simulink model "lab_2_n_4_Liza"  (R2021b)
settings: Solver=VariableStepAuto  StartTime=0.0  StopTime=100.0  RelTol=1e-3
libraries: simulink x1
settings Model: Creator=peter  LastModifiedBy=peter

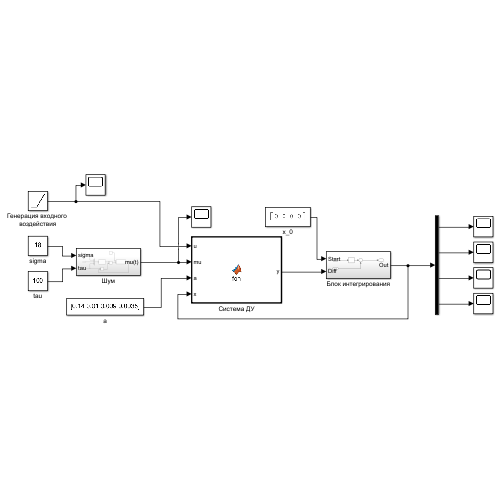
[thumbnail: Simulink's stored preview of the top-level diagram]
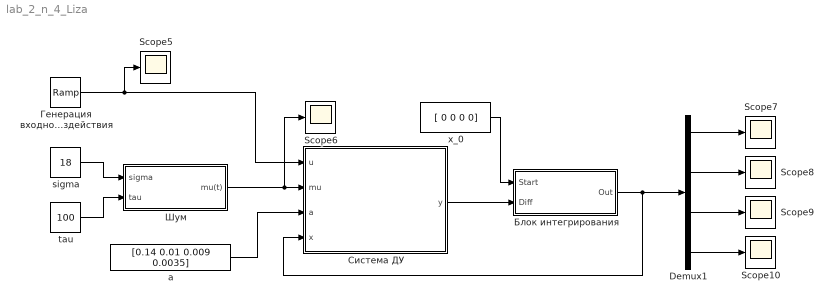
== system lab_2_n_4_Liza ==
  Demux1 : Demux
  Scope{5..10} (6 alike) : Scope
  a : Constant  Value=[0.14 0.01 0.009 0.0035]
  sigma : Constant  Value=18
  tau : Constant  Value=100
  x_0 : Constant  Value=[ 0 0 0 0]
  Блок интегрирования : Subsystem
  Генерация входного воздействия : simulink/Sources/Ramp  slope=1  start=0  InitialOutput=0
  Система ДУ : MATLAB Function  TreatAsAtomicUnit=on
  Шум : Subsystem
  wires:
  Demux1/4 -> Scope10/1
  Блок интегрирования/1(Out) -> Система ДУ/4(x), Demux1/1
  tau/1 -> Шум/2(tau)
  Система ДУ/1(y) -> Блок интегрирования/2(Diff)
  Demux1/1 -> Scope7/1
  Шум/1(mu(t)) -> Система ДУ/2(mu), Scope6/1
  a/1 -> Система ДУ/3(a)
  Генерация входного воздействия/1 -> Система ДУ/1(u), Scope5/1
  sigma/1 -> Шум/1(sigma)
  x_0/1 -> Блок интегрирования/1(Start)
  Demux1/2 -> Scope8/1
  Demux1/3 -> Scope9/1

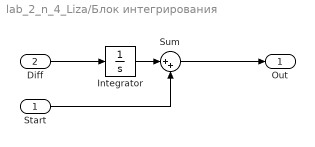
== system lab_2_n_4_Liza/Блок интегрирования ==
  Start : Inport
  Diff : Inport  Port=2
  Integrator : Integrator
  Sum : Sum  Inputs=|++
  Out : Outport
  wires:
  Diff/1 -> Integrator/1
  Sum/1 -> Out/1
  Integrator/1 -> Sum/1
  Start/1 -> Sum/2

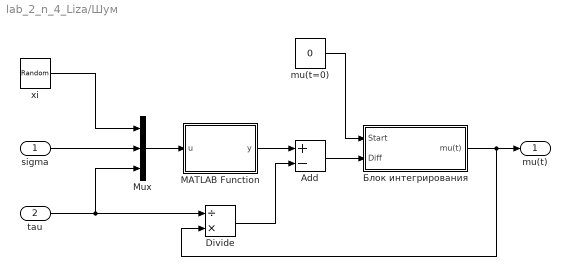
== system lab_2_n_4_Liza/Шум ==
  sigma : Inport
  tau : Inport  Port=2
  Add : Sum  Inputs=+-
  Divide : Product  Inputs=/*
  MATLAB Function : MATLAB Function  TreatAsAtomicUnit=on
  Mux : Mux  Inputs=3
  mu(t=0) : Constant  Value=0
  xi : RandomNumber  SampleTime=0.1
  Блок интегрирования : Subsystem
  mu(t) : Outport
  wires:
  mu(t=0)/1 -> Блок интегрирования/1(Start)
  Блок интегрирования/1(mu(t)) -> Divide/2, mu(t)/1
  xi/1 -> Mux/1
  sigma/1 -> Mux/2
  tau/1 -> Divide/1, Mux/3
  Add/1 -> Блок интегрирования/2(Diff)
  Divide/1 -> Add/2
  MATLAB Function/1(y) -> Add/1
  Mux/1 -> MATLAB Function/1(u)

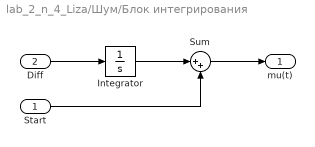
== system lab_2_n_4_Liza/Шум/Блок интегрирования ==
  Start : Inport
  Diff : Inport  Port=2
  Integrator : Integrator
  Sum : Sum  Inputs=|++
  mu(t) : Outport
  wires:
  Integrator/1 -> Sum/1
  Sum/1 -> mu(t)/1
  Diff/1 -> Integrator/1
  Start/1 -> Sum/2

== matlab function lab_2_n_4_Liza/Система ДУ ==
  data: u input; y output; mu input; a input; x input
function y = fcn(u,mu,a,x)
    dx_1=x(2);
    dx_2=x(3);
    dx_3=x(4);
    dx_4=u+mu-a(1)*x(1)-a(2)*x(2)-a(3)*x(3)-a(4)*x(4);
y = [dx_1, 
    dx_2, 
    dx_3,
    dx_4];

== matlab function lab_2_n_4_Liza/Шум/MATLAB Function ==
  data: u input; y output
function y = fcn(u)
    xi=u(1);
    sigma=u(2);
    tau=u(3);
    alpha=1/tau;
    k_f=sigma*sqrt(2*alpha);
y = k_f*xi;
